simulink model "gm_OFDM_transmitter"  (R2016b)
settings: Solver=FixedStepDiscrete  StartTime=0.0  StopTime=10  RelTol=1e-3
libraries: commdigbbndam3 x16, simulink x1, hdlsllib x1, dspxfrm3 x1
settings Model: Creator=jake  LastModifiedBy=jake
settings DataIOCC: SaveOutput=off  SaveTime=off
settings OptimizationCC: BlockReduction=off  ConditionallyExecuteInputs=off  DefaultParameterBehavior=Inlined
settings DebuggingCC: AlgebraicLoopMsg=error  InheritedTsInSrcMsg=none  SingleTaskRateTransMsg=error  StrictBusMsg=ErrorOnBusTreatedAsVector
settings HardwareCC: ProdBitPerPointer=32  ProdBitPerSizeT=32  ProdBitPerPtrDiffT=32  ProdLargestAtomicFloat=None  ProdIntDivRoundTo=Undefined  ProdEndianess=Unspecified  ProdWordSize=32  ProdHWDeviceType=ASIC/FPGA->ASIC/FPGA  ProdEqTarget=off
settings GRTTargetCC: TargetLangStandard=C89/C90 (ANSI)

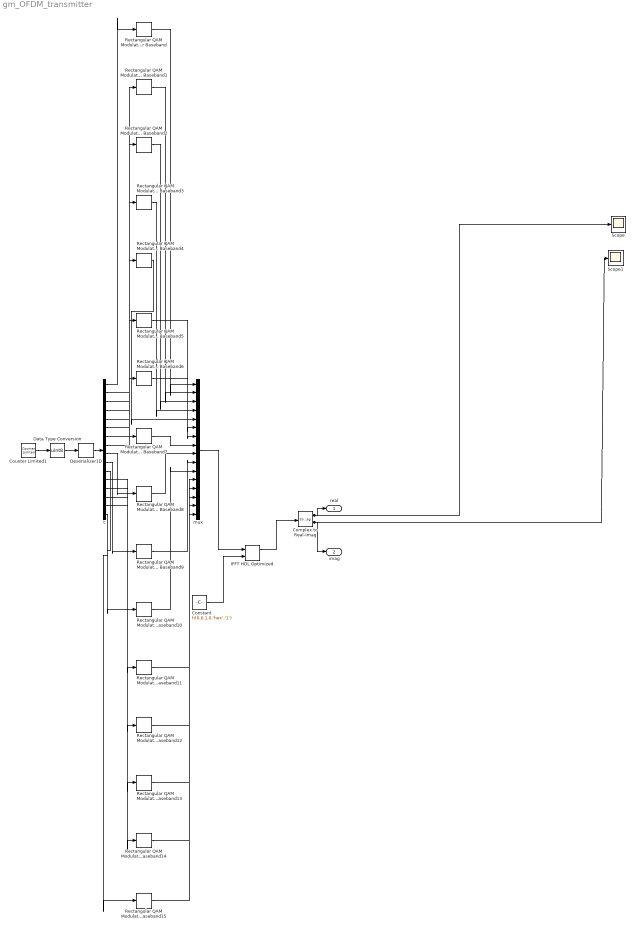
== system gm_OFDM_transmitter ==
  Complex to Real-Imag : ComplexToRealImag  SampleTime=0.32
  Constant : Constant  Value=fi(0,0,1,0,'hex','1')  OutDataTypeStr=boolean  SampleTime=-1
  Counter Limited1 : simulink/Sources/Counter Limited  uplimit=hex2num('402c000000000000')  tsamp=0.02
  Data Type Conversion : DataTypeConversion  OutDataTypeStr=uint8  SampleTime=0.02
  Deserializer1D : hdlsllib/HDL Operations/Deserializer1D  Ratio=16  IdleCycles=0  InitialCondition=fi(0,0,8,0,'hex','00')  startIn=off  validIn=off  validOut=off  inputDataDimensions=1  inputSampleTime=0.02  inputSignalType=real
  IFFT HDL Optimized : dspxfrm3/IFFT HDL Optimized  Architecture=Streaming Radix 2^2  ComplexMultiplication=Use 3 multipliers and 5 adders  BitReversedOutput=on  BitReversedInput=off  Normalize=on  FFTLength=16  SimulateUsing=Code generation  RoundingMethod=Floor  ResetInputPort=off  StartOutputPort=off  EndOutputPort=off
  Rectangular QAM Modulator Baseband{,1..15} (16 alike) : commdigbbndam3/Rectangular QAM Modulator Baseband  M=16  InType=Integer  Enc=Gray  Mapping=[0:15]  PowType=Min. distance between symbols  MinDist=2  AvgPow=1  PeakPow=1  Ph=0  outDtype=Fixed-point  outWordLen=16  outUDDataType=sfix(16)  outFracLenMode=Best precision  outFracLen=15  outDataTypeStr=fixdt(1,16)  outLastDataTypeStr=fixdt(1,16)
  Scope : Scope
  Scope1 : Scope
  mux : Mux  Inputs=16
  t : Demux  Outputs=16
  real : Outport  SignalName=ifft_real
  imag : Outport  Port=2  SignalName=ifft_imag
  wires:
  Complex to Real-Imag/1 -> Scope/1, real/1
  Complex to Real-Imag/2 -> Scope1/1, imag/1
  Constant/1 -> IFFT HDL Optimized/2
  Counter Limited1/1 -> Data Type Conversion/1
  Data Type Conversion/1 -> Deserializer1D/1
  Deserializer1D/1 -> t/1
  IFFT HDL Optimized/1 -> Complex to Real-Imag/1
  mux/1 -> IFFT HDL Optimized/1
  Rectangular QAM Modulator Baseband/1 -> mux/1
  Rectangular QAM Modulator Baseband1/1 -> mux/2
  Rectangular QAM Modulator Baseband10/1 -> mux/11
  Rectangular QAM Modulator Baseband11/1 -> mux/12
  Rectangular QAM Modulator Baseband12/1 -> mux/13
  Rectangular QAM Modulator Baseband13/1 -> mux/14
  Rectangular QAM Modulator Baseband14/1 -> mux/15
  Rectangular QAM Modulator Baseband15/1 -> mux/16
  Rectangular QAM Modulator Baseband2/1 -> mux/3
  Rectangular QAM Modulator Baseband3/1 -> mux/4
  Rectangular QAM Modulator Baseband4/1 -> mux/5
  Rectangular QAM Modulator Baseband5/1 -> mux/6
  Rectangular QAM Modulator Baseband6/1 -> mux/7
  Rectangular QAM Modulator Baseband7/1 -> mux/8
  Rectangular QAM Modulator Baseband8/1 -> mux/9
  Rectangular QAM Modulator Baseband9/1 -> mux/10
  t/1 -> Rectangular QAM Modulator Baseband/1
  t/2 -> Rectangular QAM Modulator Baseband1/1
  t/3 -> Rectangular QAM Modulator Baseband2/1
  t/4 -> Rectangular QAM Modulator Baseband3/1
  t/5 -> Rectangular QAM Modulator Baseband4/1
  t/6 -> Rectangular QAM Modulator Baseband5/1
  t/7 -> Rectangular QAM Modulator Baseband6/1
  t/8 -> Rectangular QAM Modulator Baseband7/1
  t/9 -> Rectangular QAM Modulator Baseband8/1
  t/10 -> Rectangular QAM Modulator Baseband9/1
  t/11 -> Rectangular QAM Modulator Baseband10/1
  t/12 -> Rectangular QAM Modulator Baseband11/1
  t/13 -> Rectangular QAM Modulator Baseband12/1
  t/14 -> Rectangular QAM Modulator Baseband13/1
  t/15 -> Rectangular QAM Modulator Baseband14/1
  t/16 -> Rectangular QAM Modulator Baseband15/1
